simulink model "ex2"  (R2020a)
settings: Solver=FixedStepAuto  StartTime=0.0  StopTime=10.0  FixedStep=0.05  RelTol=1e-3
libraries: simulink x1

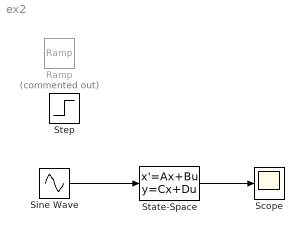
== system ex2 ==
  Ramp : simulink/Sources/Ramp  Commented=on  slope=1  start=0  InitialOutput=0
  Scope : Scope
  Sine Wave : Sin  Frequency=2*pi  SampleTime=0
  State-Space : StateSpace  A=[0 1 0;0 0 1;-6 -11 -6]  B=[1; 1; 1]  C=[1 1 0]  D=[0]  InitialCondition=[1;0.5;-0.5]
  Step : Step  SampleTime=0
  wires:
  State-Space/1 -> Scope/1
  Sine Wave/1 -> State-Space/1
